simulink model "Fixed_point"  (R2022b)
settings: Solver=VariableStepAuto  StartTime=0.0  StopTime=10.0  RelTol=1e-3
settings Model: Creator=Sonikot  LastModifiedBy=Sonikot

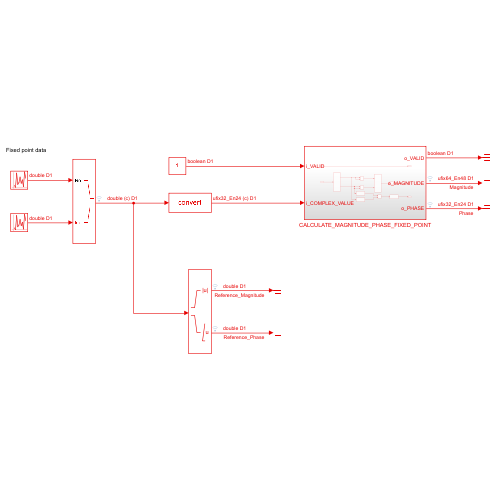
[thumbnail: Simulink's stored preview of the top-level diagram]
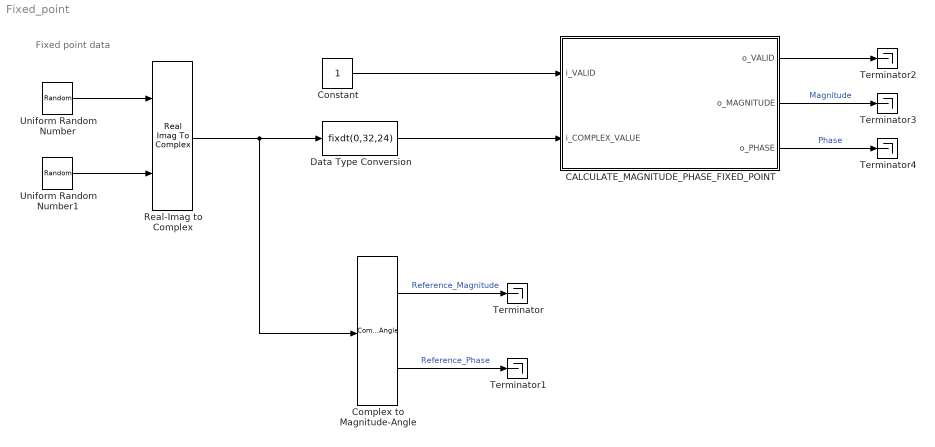
== system Fixed_point ==
  note: Fixed point data
  CALCULATE_MAGNITUDE_PHASE_FIXED_POINT : Subsystem
  Complex to Magnitude-Angle : ComplexToMagnitudeAngle
  Constant : Constant  OutDataTypeStr=boolean  SampleTime=1
  Data Type Conversion : DataTypeConversion  OutDataTypeStr=fixdt(0,32,24)  RndMeth=Round  SaturateOnIntegerOverflow=off
  Real-Imag to Complex : RealImagToComplex
  Terminator{,1..4} (5 alike) : Terminator
  Uniform Random Number : UniformRandomNumber  Minimum=0  Maximum=255.99999994039535522461  Seed=8  SampleTime=1
  Uniform Random Number1 : UniformRandomNumber  Minimum=0  Maximum=255.99999994039535522461  Seed=9  SampleTime=1
  wires:
  Uniform Random Number/1 -> Real-Imag to Complex/1
  Uniform Random Number1/1 -> Real-Imag to Complex/2
  Real-Imag to Complex/1 -> Complex to Magnitude-Angle/1, Data Type Conversion/1
  Constant/1 -> CALCULATE_MAGNITUDE_PHASE_FIXED_POINT/1(i_VALID)
  Data Type Conversion/1 -> CALCULATE_MAGNITUDE_PHASE_FIXED_POINT/2(i_COMPLEX_VALUE)
  Complex to Magnitude-Angle/1 -> Terminator/1  "Reference_Magnitude"
  Complex to Magnitude-Angle/2 -> Terminator1/1  "Reference_Phase"
  CALCULATE_MAGNITUDE_PHASE_FIXED_POINT/1(o_VALID) -> Terminator2/1
  CALCULATE_MAGNITUDE_PHASE_FIXED_POINT/2(o_MAGNITUDE) -> Terminator3/1  "Magnitude"
  CALCULATE_MAGNITUDE_PHASE_FIXED_POINT/3(o_PHASE) -> Terminator4/1  "Phase"

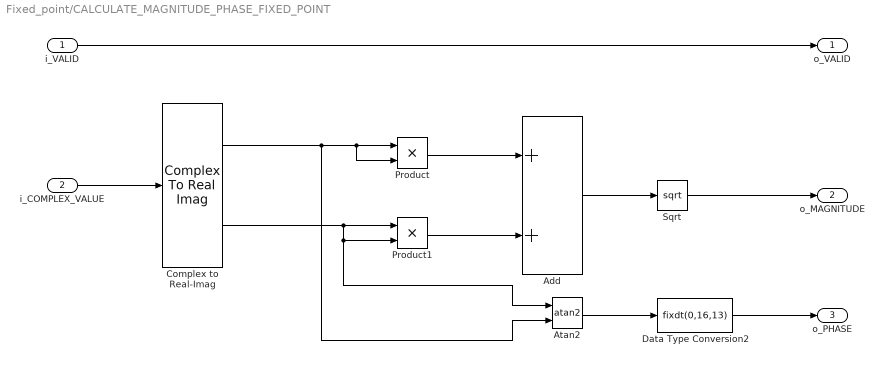
== system Fixed_point/CALCULATE_MAGNITUDE_PHASE_FIXED_POINT ==
  i_VALID : Inport
  i_COMPLEX_VALUE : Inport  Port=2
  Add : Sum  OutDataTypeStr=fixdt(0,65,48)
  Atan2 : Trigonometry  Operator=atan2  ApproximationMethod=CORDIC  NumberOfIterations=20
  Complex to Real-Imag : ComplexToRealImag
  Data Type Conversion2 : DataTypeConversion  OutDataTypeStr=fixdt(0,16,13)  SaturateOnIntegerOverflow=off  RndMeth=Floor
  Product : Product
  Product1 : Product
  Sqrt : Sqrt  OutDataTypeStr=fixdt(0,33,24 )
  o_VALID : Outport
  o_MAGNITUDE : Outport  Port=2
  o_PHASE : Outport  Port=3
  wires:
  Sqrt/1 -> o_MAGNITUDE/1
  i_VALID/1 -> o_VALID/1
  Add/1 -> Sqrt/1
  i_COMPLEX_VALUE/1 -> Complex to Real-Imag/1
  Product1/1 -> Add/2
  Product/1 -> Add/1
  Complex to Real-Imag/2 -> Product1/1, Atan2/1, Product1/2
  Complex to Real-Imag/1 -> Atan2/2, Product/2, Product/1
  Atan2/1 -> Data Type Conversion2/1
  Data Type Conversion2/1 -> o_PHASE/1
